simulink model "gm_CustArch_v5_vnl"  (R2020a)
settings: Solver=FixedStepDiscrete  StartTime=0.0  StopTime=840000  RelTol=1e-3
libraries: simulink x179, hdlsllib x113
(part 3 of 4)

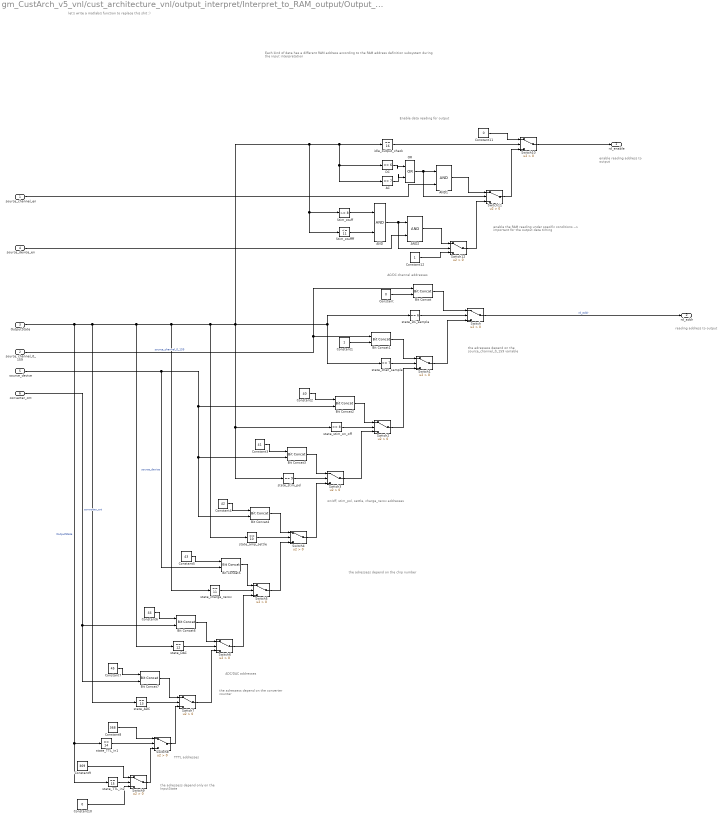
== system gm_CustArch_v5_vnl/cust_architecture_vnl/output_interpret/Interpret_to_RAM_output/Output_State_to_RAM_address (to read) ==
  note: enable reading address
      | to output
  note: Each kind of data has a different RAM
      | address according to the
      | RAM address definition subsystem during the
      | input interpretation
  note: the adressess depend on the
      | source_channel_0_159 variable
  note: AC/DC channel addresses
  note: ADC/DAC addresses
  note: on/off, stim_pol, settle, charge_recov addresses
  note: the adressess depend on the converter
      | counter
  note: the adressess depend only on the
      | InputState
  note: the adressess depend on the chip number
  note: TTTL addresses
  note: let's write a matlab/s function to replace this shit :)
  note: Enable data reading for output
  note: enable the RAM reading under specific conditions
      | --> important for the output data timing
  note: reading address
      | to output
  source_channel_en : Inport
  source_channel_0_159 : Inport  Port=2
  OutputState : Inport  Port=3
  source_device_en : Inport  Port=4
  source_device : Inport  Port=5
  converter_cnt : Inport  Port=6
  AC : simulink/Logic and Bit Operations/Compare To Constant  relop===  const=7  OutDataTypeStr=boolean
  AND : Logic  IconShape=distinctive  AllPortsSameDT=off  OutDataTypeStr=boolean
  AND1 : Logic  IconShape=distinctive  AllPortsSameDT=off  OutDataTypeStr=boolean
  AND2 : Logic  IconShape=distinctive  AllPortsSameDT=off  OutDataTypeStr=boolean
  Bit Concat{,1..7} (8 alike) : hdlsllib/Logic and Bit Operations/Bit Concat  numInputs=2
  Constant : Constant  Value=0  OutDataTypeStr=boolean  SampleTime=-1
  Constant1 : Constant  OutDataTypeStr=boolean  SampleTime=-1
  Constant10 : Constant  Value=0  OutDataTypeStr=fixdt(0,9)  SampleTime=-1
  Constant11 : Constant  Value=0  OutDataTypeStr=boolean  SampleTime=-1
  Constant12 : Constant  OutDataTypeStr=boolean  SampleTime=-1
  Constant2 : Constant  Value=40  OutDataTypeStr=fixdt(0,6)  SampleTime=-1
  Constant3 : Constant  Value=41  OutDataTypeStr=fixdt(0,6)  SampleTime=-1
  Constant4 : Constant  Value=42  OutDataTypeStr=fixdt(0,6)  SampleTime=-1
  Constant5 : Constant  Value=43  OutDataTypeStr=fixdt(0,6)  SampleTime=-1
  Constant6 : Constant  Value=44  OutDataTypeStr=fixdt(0,6)  SampleTime=-1
  Constant7 : Constant  Value=45  OutDataTypeStr=fixdt(0,6)  SampleTime=-1
  Constant8 : Constant  Value=368  OutDataTypeStr=fixdt(0,9)  SampleTime=-1
  Constant9 : Constant  Value=369  OutDataTypeStr=fixdt(0,9)  SampleTime=-1
  DC : simulink/Logic and Bit Operations/Compare To Constant  relop===  const=6  OutDataTypeStr=boolean
  OR : Logic  Operator=OR  IconShape=distinctive  AllPortsSameDT=off  OutDataTypeStr=boolean
  Stim_stuff : simulink/Logic and Bit Operations/Compare To Constant  relop=>=  const=8  OutDataTypeStr=boolean
  Stim_stuffff : simulink/Logic and Bit Operations/Compare To Constant  relop=<=  const=11  OutDataTypeStr=boolean
  Switch{,1..12} (13 alike) : Switch  Criteria=u2 > Threshold
  idle_output_check : simulink/Logic and Bit Operations/Compare To Constant  relop===  const=16  OutDataTypeStr=boolean
  state_ADC : simulink/Logic and Bit Operations/Compare To Constant  relop===  const=13  OutDataTypeStr=boolean
  state_DAC : simulink/Logic and Bit Operations/Compare To Constant  relop===  const=12  OutDataTypeStr=boolean
  state_DC_sample : simulink/Logic and Bit Operations/Compare To Constant  relop===  const=6  OutDataTypeStr=boolean
  state_TTL_in1 : simulink/Logic and Bit Operations/Compare To Constant  relop===  const=14  OutDataTypeStr=boolean
  state_TTL_in2 : simulink/Logic and Bit Operations/Compare To Constant  relop===  const=15  OutDataTypeStr=boolean
  state_amp_settle : simulink/Logic and Bit Operations/Compare To Constant  relop===  const=10  OutDataTypeStr=boolean
  state_chan_sample : simulink/Logic and Bit Operations/Compare To Constant  relop===  const=7  OutDataTypeStr=boolean
  state_charge_recov : simulink/Logic and Bit Operations/Compare To Constant  relop===  const=11  OutDataTypeStr=boolean
  state_stim_on_off : simulink/Logic and Bit Operations/Compare To Constant  relop===  const=8  OutDataTypeStr=boolean
  state_stim_pol : simulink/Logic and Bit Operations/Compare To Constant  relop===  const=9  OutDataTypeStr=boolean
  rd_enable : Outport  VectorParamsAs1DForOutWhenUnconnected=off
  rd_addr : Outport  Port=2  OutDataTypeStr=fixdt(0,9,0)  VectorParamsAs1DForOutWhenUnconnected=off
  wires:
  Switch10/1 -> rd_enable/1
  Constant12/1 -> Switch12/3
  Switch12/1 -> Switch11/3
  AND2/1 -> Switch12/1
  AND1/1 -> Switch11/1
  Switch11/1 -> Switch10/3
  Constant11/1 -> Switch10/1
  source_device_en/1 -> AND2/2
  source_channel_en/1 -> AND1/2
  AND/1 -> AND2/1, Switch12/2
  Stim_stuffff/1 -> AND/2
  Stim_stuff/1 -> AND/1
  idle_output_check/1 -> Switch10/2
  OR/1 -> AND1/1, Switch11/2
  AC/1 -> OR/2
  DC/1 -> OR/1
  Constant10/1 -> Switch9/3
  Switch9/1 -> Switch8/3
  Constant9/1 -> Switch9/1
  state_TTL_in2/1 -> Switch9/2
  Switch8/1 -> Switch7/3
  OutputState/1 -> state_ADC/1, state_charge_recov/1, Stim_stuff/1, Stim_stuffff/1, idle_output_check/1, DC/1, AC/1, state_chan_sample/1, state_DC_sample/1, state_stim_on_off/1, state_stim_pol/1, state_amp_settle/1, state_DAC/1, state_TTL_in1/1, state_TTL_in2/1  "OutputState"
  Constant8/1 -> Switch8/1
  state_TTL_in1/1 -> Switch8/2
  Switch7/1 -> Switch6/3
  Constant7/1 -> Bit Concat7/1
  state_ADC/1 -> Switch7/2
  Bit Concat7/1 -> Switch7/1
  converter_cnt/1 -> Bit Concat6/2, Bit Concat7/2  "converter_cnt"
  Switch6/1 -> Switch5/3
  Constant6/1 -> Bit Concat6/1
  state_DAC/1 -> Switch6/2
  Bit Concat6/1 -> Switch6/1
  Switch5/1 -> Switch4/3
  source_device/1 -> Bit Concat2/2, Bit Concat3/2, Bit Concat4/2, Bit Concat5/2  "source_device"
  Constant5/1 -> Bit Concat5/1
  state_charge_recov/1 -> Switch5/2
  Bit Concat5/1 -> Switch5/1
  Switch4/1 -> Switch3/3
  Bit Concat4/1 -> Switch4/1
  state_amp_settle/1 -> Switch4/2
  Constant4/1 -> Bit Concat4/1
  Switch3/1 -> Switch2/3
  Bit Concat3/1 -> Switch3/1
  state_stim_pol/1 -> Switch3/2
  Constant3/1 -> Bit Concat3/1
  Switch2/1 -> Switch1/3
  state_stim_on_off/1 -> Switch2/2
  Bit Concat2/1 -> Switch2/1
  Constant2/1 -> Bit Concat2/1
  Switch/1 -> rd_addr/1  "rd_addr"
  Switch1/1 -> Switch/3
  Bit Concat1/1 -> Switch1/1
  Constant1/1 -> Bit Concat1/2
  state_chan_sample/1 -> Switch1/2
  Bit Concat/1 -> Switch/1
  Constant/1 -> Bit Concat/2
  source_channel_0_159/1 -> Bit Concat/1, Bit Concat1/1  "source_channel_0_159"
  state_DC_sample/1 -> Switch/2

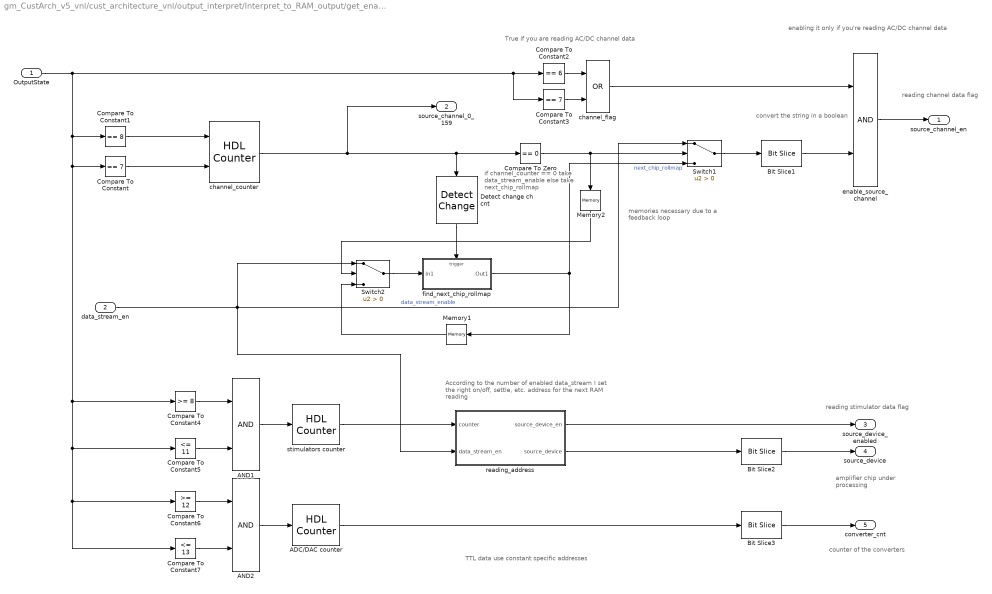
== system gm_CustArch_v5_vnl/cust_architecture_vnl/output_interpret/Interpret_to_RAM_output/get_enabled_timings  ==
  note: counter of the converters
  note: reading stimulator data flag
  note: TTL data use constant specific addresses
  note: enabling it only if you're reading AC/DC channel data
  note: True if you are reading AC/DC channel data
  note: convert the string
      | in a boolean
  note: According to the number of enabled data_stream
      | I set the right on/off, settle, etc. address for the next
      | RAM reading
  note: amplifier chip under
      | processing
  note: if channel_counter == 0
      | take data_stream_enable
      | else take next_chip_rollmap
  note: memories necessary due to
      | a feedback loop
  note: reading channel data flag
  OutputState : Inport
  data_stream_en : Inport  Port=2
  ADC/DAC counter : hdlsllib/Sources/HDL Counter  CountType=Count limited  CountInit=0  CountStep=1  CountMax=7  CountFromType=Specify  CountFrom=0  CountResetPort=off  CountLoadPort=off  CountEnbPort=on  CountDirPort=off  CountDataType=Unsigned  CountWordLen=8  CountFracLen=0  CountSampTime=1
  AND1 : Logic  IconShape=distinctive  AllPortsSameDT=off  OutDataTypeStr=boolean
  AND2 : Logic  IconShape=distinctive  AllPortsSameDT=off  OutDataTypeStr=boolean
  Bit Slice1 : hdlsllib/Logic and Bit Operations/Bit Slice  lidx=0  ridx=0
      settings: SourceProductBaseCode=SL
  Bit Slice2 : hdlsllib/Logic and Bit Operations/Bit Slice  lidx=2  ridx=0
      settings: SourceProductBaseCode=SL
  Bit Slice3 : hdlsllib/Logic and Bit Operations/Bit Slice  lidx=2  ridx=0
      settings: SourceProductBaseCode=SL
  Compare To Constant : simulink/Logic and Bit Operations/Compare To Constant  relop===  const=7  OutDataTypeStr=boolean
  Compare To Constant1 : simulink/Logic and Bit Operations/Compare To Constant  relop===  const=8  OutDataTypeStr=boolean
  Compare To Constant2 : simulink/Logic and Bit Operations/Compare To Constant  relop===  const=6  OutDataTypeStr=boolean
  Compare To Constant3 : simulink/Logic and Bit Operations/Compare To Constant  relop===  const=7  OutDataTypeStr=boolean
  Compare To Constant4 : simulink/Logic and Bit Operations/Compare To Constant  relop=>=  const=8  OutDataTypeStr=boolean
  Compare To Constant5 : simulink/Logic and Bit Operations/Compare To Constant  relop=<=  const=11  OutDataTypeStr=boolean
  Compare To Constant6 : simulink/Logic and Bit Operations/Compare To Constant  relop=>=  const=12  OutDataTypeStr=boolean
  Compare To Constant7 : simulink/Logic and Bit Operations/Compare To Constant  relop=<=  const=13  OutDataTypeStr=boolean
  Compare To Zero : simulink/Logic and Bit Operations/Compare To Zero  relop===  OutDataTypeStr=boolean
  Detect change ch cnt : simulink/Logic and Bit Operations/Detect Change  vinit=0  OutDataTypeStr=boolean
  Memory1 : Memory  InheritSampleTime=on
  Memory2 : Memory  InheritSampleTime=on
  Switch1 : Switch  Criteria=u2 > Threshold
  Switch2 : Switch  Criteria=u2 > Threshold
  channel_counter : hdlsllib/Sources/HDL Counter  CountType=Count limited  CountInit=0  CountStep=1  CountMax=159  CountFromType=Specify  CountFrom=0  CountResetPort=on  CountLoadPort=off  CountEnbPort=on  CountDirPort=off  CountDataType=Unsigned  CountWordLen=8  CountFracLen=0  CountSampTime=1
  channel_flag : Logic  Operator=OR  IconShape=distinctive  AllPortsSameDT=off  OutDataTypeStr=boolean
  enable_source_channel : Logic  IconShape=distinctive  AllPortsSameDT=off  OutDataTypeStr=boolean
  find_next_chip_rollmap : Subsystem  TreatAsAtomicUnit=on
  reading_address : Subsystem
  stimulators counter : hdlsllib/Sources/HDL Counter  CountType=Count limited  CountInit=0  CountStep=1  CountMax=7  CountFromType=Specify  CountFrom=0  CountResetPort=off  CountLoadPort=off  CountEnbPort=on  CountDirPort=off  CountDataType=Unsigned  CountWordLen=8  CountFracLen=0  CountSampTime=1
  source_channel_en : Outport  VectorParamsAs1DForOutWhenUnconnected=off
  source_channel_0_159 : Outport  Port=2  OutMin=0  OutMax=159  OutDataTypeStr=uint8  VectorParamsAs1DForOutWhenUnconnected=off  LockScale=on
  source_device_enabled : Outport  Port=3  VectorParamsAs1DForOutWhenUnconnected=off
  source_device : Outport  Port=4  VectorParamsAs1DForOutWhenUnconnected=off
  converter_cnt : Outport  Port=5  VectorParamsAs1DForOutWhenUnconnected=off
  wires:
  Compare To Constant/1 -> channel_counter/2
  Compare To Constant1/1 -> channel_counter/1
  ADC/DAC counter/1 -> Bit Slice3/1
  AND2/1 -> ADC/DAC counter/1
  Compare To Constant7/1 -> AND2/2
  OutputState/1 -> Compare To Constant2/1, Compare To Constant3/1, Compare To Constant4/1, Compare To Constant5/1, Compare To Constant7/1, Compare To Constant6/1, Compare To Constant/1, Compare To Constant1/1
  Bit Slice3/1 -> converter_cnt/1
  Compare To Constant6/1 -> AND2/1
  data_stream_en/1 -> Switch2/1, reading_address/2(data_stream_en), Switch1/1  "data_stream_enable"
  reading_address/2(source_device) -> Bit Slice2/1
  stimulators counter/1 -> reading_address/1("counter ")
  AND1/1 -> stimulators counter/1
  Bit Slice2/1 -> source_device/1
  reading_address/1(source_device_en) -> source_device_enabled/1
  Compare To Constant5/1 -> AND1/2
  Compare To Constant4/1 -> AND1/1
  Bit Slice1/1 -> enable_source_channel/2
  Switch1/1 -> Bit Slice1/1
  enable_source_channel/1 -> source_channel_en/1
  channel_flag/1 -> enable_source_channel/1
  Compare To Constant2/1 -> channel_flag/1
  Compare To Constant3/1 -> channel_flag/2
  Memory2/1 -> Switch2/2
  Compare To Zero/1 -> Memory2/1, Switch1/2
  Switch2/1 -> find_next_chip_rollmap/1(In1)
  Memory1/1 -> Switch2/3
  find_next_chip_rollmap/1(Out1) -> Switch1/3, Memory1/1  "next_chip_rollmap"
  Detect change ch cnt/1 -> find_next_chip_rollmap/Trigger
  channel_counter/1 -> source_channel_0_159/1, Compare To Zero/1, Detect change ch cnt/1

== system gm_CustArch_v5_vnl/cust_architecture_vnl/process_and_retrieve/digital_filter/HP_Butter_1st ==
  Input : Inport  OutDataTypeStr=fixdt(1,16,4)
  Input1 : Inport  Port=2  OutDataTypeStr=fixdt(1,16,2)
  CastState1 : DataTypeConversion  OutDataTypeStr=fixdt(1,16,2)  RndMeth=Convergent  SaturateOnIntegerOverflow=on
  ConvertIn : DataTypeConversion  OutDataTypeStr=fixdt(1,16,4)  RndMeth=Nearest  SaturateOnIntegerOverflow=on
  ConvertOut : DataTypeConversion  OutDataTypeStr=fixdt(1,16,5)  RndMeth=Convergent  SaturateOnIntegerOverflow=on
  SumA21 : Sum  Inputs=|+-  AccumDataTypeStr=fixdt(1,34,20)  OutDataTypeStr=fixdt(1,34,20)  RndMeth=Convergent  SaturateOnIntegerOverflow=on
  SumB21 : Sum  Inputs=|+-  AccumDataTypeStr=fixdt(1,34,20)  OutDataTypeStr=fixdt(1,34,23)  RndMeth=Convergent  SaturateOnIntegerOverflow=on
  a(2)(1) : Gain  Gain=-0.939062505817492399  ParamDataTypeStr=fixdt(1,16,15)  OutDataTypeStr=fixdt(1,32,18)  RndMeth=Convergent  SaturateOnIntegerOverflow=on
  s(1) : Gain  Gain=0.969531252908746199  ParamDataTypeStr=fixdt(0,16,16)  OutDataTypeStr=fixdt(1,16,4)  RndMeth=Convergent  SaturateOnIntegerOverflow=on
  Output : Outport
  Output1 : Outport  Port=2
  wires:
  Input1/1 -> a(2)(1)/1, SumB21/2
  ConvertIn/1 -> s(1)/1
  ConvertOut/1 -> Output/1
  CastState1/1 -> SumB21/1, Output1/1
  a(2)(1)/1 -> SumA21/2
  SumB21/1 -> ConvertOut/1
  SumA21/1 -> CastState1/1
  s(1)/1 -> SumA21/1
  Input/1 -> ConvertIn/1

== system gm_CustArch_v5_vnl/cust_architecture_vnl/process_and_retrieve/previous_sample_storage/PreviousData_read ==
  u2 : Inport
  Enable : EnablePort
  1st1 : Constant  OutDataTypeStr=boolean  SampleTime=-1
  Bit Concat1 : hdlsllib/Logic and Bit Operations/Bit Concat  numInputs=2
  y : Outport  InitialOutput=[0]
  wires:
  Bit Concat1/1 -> y/1
  1st1/1 -> Bit Concat1/1
  u2/1 -> Bit Concat1/2

== system gm_CustArch_v5_vnl/cust_architecture_vnl/process_and_retrieve/previous_sample_storage1/PreviousData_read ==
  u2 : Inport
  Enable : EnablePort  StatesWhenEnabling=reset
  1st1 : Constant  OutDataTypeStr=boolean  SampleTime=-1
  Bit Concat1 : hdlsllib/Logic and Bit Operations/Bit Concat  numInputs=2
  y : Outport  OutputWhenDisabled=reset  InitialOutput=[0]
  wires:
  Bit Concat1/1 -> y/1
  1st1/1 -> Bit Concat1/1
  u2/1 -> Bit Concat1/2

== system gm_CustArch_v5_vnl/cust_architecture/input_interpret_store_retrieve/Interpret_to_RAM_input/interpret incoming data/condition to count DAC or ADC  ==
  fifo_write_to : Inport  OutDataTypeStr=boolean  PortDimensions=1  SampleTime=1
  input_state : Inport  Port=2  OutDataTypeStr=uint8  PortDimensions=1  SampleTime=1
  AND : Logic  AllPortsSameDT=off  OutDataTypeStr=boolean  SampleTime=1
  OR : Logic  Operator=OR  AllPortsSameDT=off  OutDataTypeStr=boolean  SampleTime=1
  is state_ADC : simulink/Logic and Bit Operations/Compare To Constant  relop===  const="fi(0,0,8,0,\"hex\",\"0d\")"  OutDataTypeStr=boolean
  is state_DAC : simulink/Logic and Bit Operations/Compare To Constant  relop===  const="fi(0,0,8,0,\"hex\",\"0c\")"  OutDataTypeStr=boolean
  Out1 : Outport  VectorParamsAs1DForOutWhenUnconnected=off
  wires:
  is state_DAC/1 -> OR/1
  is state_ADC/1 -> OR/2
  OR/1 -> AND/2
  AND/1 -> Out1/1
  input_state/1 -> is state_ADC/1, is state_DAC/1
  fifo_write_to/1 -> AND/1

== system gm_CustArch_v5_vnl/cust_architecture/input_interpret_store_retrieve/Interpret_to_RAM_input/interpret incoming data/get_sources_and_RAM_addresses ==
  note: necessary to move forward from state 6 to 8
  note: 0-159 --> 20 (16 electrodes + 4 aux commands) x 8 chips
  note: if next_chip_rollmap == 00000000 I have cycled among all the chip so let's restart from data_stream_enable
  note: the data_stream_enable is a 8-bit string in which if a bit is 1 the data stream of that chip is enabled
  note: TTL data use constant specific addresses
  FIFO_write_to : Inport  OutDataTypeStr=boolean  PortDimensions=1  SampleTime=1
  InputState : Inport  Port=2  OutDataTypeStr=uint8  PortDimensions=1  SampleTime=1
  data_stream_enable : Inport  Port=3  OutDataTypeStr=uint8  PortDimensions=1  SampleTime=1
  AND1 : Logic  AllPortsSameDT=off  OutDataTypeStr=boolean  SampleTime=1
  AND2 : Logic  AllPortsSameDT=off  OutDataTypeStr=boolean  SampleTime=1
  AND3 : Logic  AllPortsSameDT=off  OutDataTypeStr=boolean  SampleTime=1
  Compare To Constant1 : simulink/Logic and Bit Operations/Compare To Constant  relop===  const="fi(0,0,8,0,\"hex\",\"00\")"  OutDataTypeStr=boolean
  Compare To Constant2 : simulink/Logic and Bit Operations/Compare To Constant  relop===  const="fi(0,0,8,0,\"hex\",\"0d\")"  OutDataTypeStr=boolean
  Compare To Constant3 : simulink/Logic and Bit Operations/Compare To Constant  relop===  const="fi(0,0,8,0,\"hex\",\"06\")"  OutDataTypeStr=boolean
  Compare To Constant4 : simulink/Logic and Bit Operations/Compare To Constant  relop=>=  const="fi(0,0,8,0,\"hex\",\"08\")"  OutDataTypeStr=boolean
  Compare To Constant5 : simulink/Logic and Bit Operations/Compare To Constant  relop===  const="fi(0,0,8,0,\"hex\",\"00\")"  OutDataTypeStr=boolean
  Compare To Constant6 : simulink/Logic and Bit Operations/Compare To Constant  relop=<=  const="fi(0,0,8,0,\"hex\",\"0b\")"  OutDataTypeStr=boolean
  Memory : UnitDelay  InitialCondition=double(0)  SampleTime=1
  Memory1 : UnitDelay  InitialCondition=double(0)  SampleTime=1
  Memory2 : UnitDelay  InitialCondition=double(0)  SampleTime=1
  OR : Logic  Operator=OR  AllPortsSameDT=off  OutDataTypeStr=boolean  SampleTime=1
  RAM_address_channel_data : Subsystem
  Switch : Switch  Criteria=u2 > Threshold  Threshold=double(0)  OutDataTypeStr=uint8  SampleTime=1
  Switch1 : Switch  Criteria=u2 > Threshold  Threshold=double(0)  OutDataTypeStr=uint8  SampleTime=1
  channel_counter : hdlsllib/Sources/HDL Counter  CountType=Count limited  CountInit=double(0)  CountStep=double(1)  CountMax=double(20)  CountFromType=Initial value  CountFrom=double(0)  CountResetPort=on  CountLoadPort=off  CountEnbPort=on  CountDirPort=off  CountDataType=Unsigned  CountWordLen=8  CountFracLen=0  CountSampTime=1
  enable_RAM_indexing : Logic  AllPortsSameDT=off  OutDataTypeStr=boolean  SampleTime=1
  enable_source_chip_transmission : Subsystem
  find_first_one_pos : Subsystem
  find_next_chip_rollmap : Subsystem
  source_device : Outport  VectorParamsAs1DForOutWhenUnconnected=off
  device_output : Outport  Port=2  VectorParamsAs1DForOutWhenUnconnected=off
  source_channel : Outport  Port=3  VectorParamsAs1DForOutWhenUnconnected=off
  inc_source_device : Outport  Port=4  VectorParamsAs1DForOutWhenUnconnected=off
  wires:
  find_next_chip_rollmap/1(bit_masked) -> Memory/1, Compare To Constant5/1
  find_first_one_pos/1(first_one_pos) -> find_next_chip_rollmap/2(source_chip), enable_source_chip_transmission/1(In1)
  enable_source_chip_transmission/1(Out1) -> RAM_address_channel_data/1(source_device), source_device/1
  enable_RAM_indexing/1 -> find_first_one_pos/Enable, find_next_chip_rollmap/Enable, RAM_address_channel_data/Enable, enable_source_chip_transmission/Enable, Memory2/1, AND2/1
  channel_counter/1 -> RAM_address_channel_data/2(dev_output), device_output/1
  Switch1/1 -> Switch/3
  Switch/1 -> find_first_one_pos/1(In1), find_next_chip_rollmap/1(curr_chip_rollmap)
  RAM_address_channel_data/1(source_channel_0_159) -> source_channel/1
  OR/1 -> enable_RAM_indexing/2
  Memory2/1 -> AND3/2
  Memory1/1 -> AND3/1, Switch1/2
  Memory/1 -> Switch1/3
  Compare To Constant6/1 -> AND1/2
  Compare To Constant5/1 -> Memory1/1, AND2/2
  Compare To Constant4/1 -> AND1/1
  Compare To Constant3/1 -> OR/1
  Compare To Constant2/1 -> channel_counter/1
  Compare To Constant1/1 -> Switch/2
  AND3/1 -> channel_counter/2
  AND2/1 -> inc_source_device/1
  AND1/1 -> OR/2
  data_stream_enable/1 -> Switch/1, Switch1/1
  InputState/1 -> Compare To Constant1/1, Compare To Constant2/1, Compare To Constant3/1, Compare To Constant4/1, Compare To Constant6/1
  FIFO_write_to/1 -> enable_RAM_indexing/1

== system gm_CustArch_v5_vnl/cust_architecture/output_interpret/Interpret_to_RAM_output/get_enabled_timings /find_next_chip_rollmap ==
  In1 : Inport  OutDataTypeStr=uint8  PortDimensions=1
  Trigger : TriggerPort  VariantControl=(inherit)  PortDimensions=1  OutDataTypeStr=boolean
  Bit Rotate : hdlsllib/Logic and Bit Operations/Bit Rotate  mode=Rotate Right  N=double(1)
      settings: SourceProductBaseCode=SL
  Out1 : Outport  InitialOutput=0  VectorParamsAs1DForOutWhenUnconnected=off
  wires:
  Bit Rotate/1 -> Out1/1
  In1/1 -> Bit Rotate/1

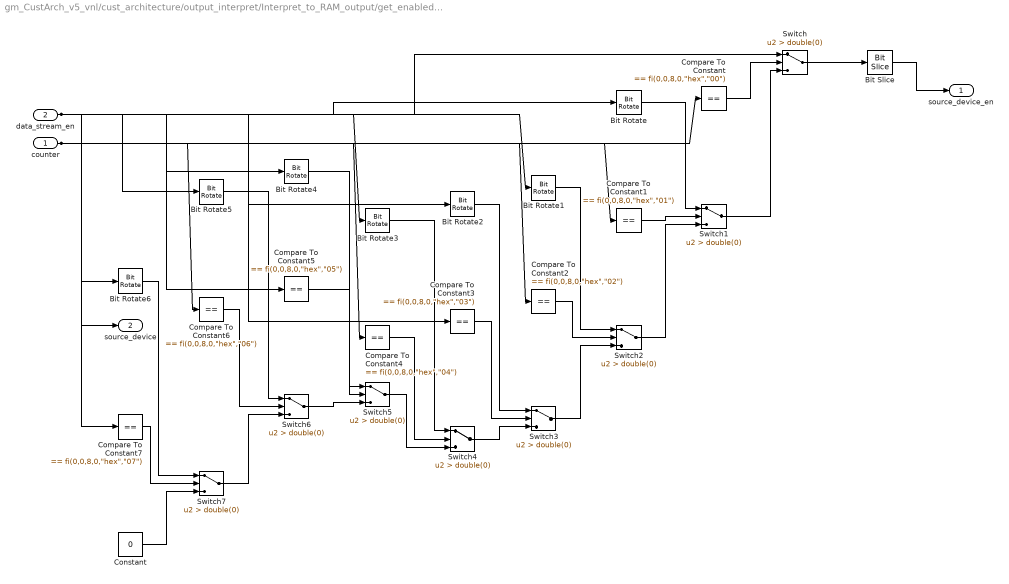
== system gm_CustArch_v5_vnl/cust_architecture/output_interpret/Interpret_to_RAM_output/get_enabled_timings /reading_address ==
  "counter " : Inport  OutDataTypeStr=uint8  PortDimensions=1  SampleTime=1
  data_stream_en : Inport  Port=2  OutDataTypeStr=uint8  PortDimensions=1  SampleTime=1
  Bit Rotate : hdlsllib/Logic and Bit Operations/Bit Rotate  mode=Rotate Right  N=double(1)
      settings: SourceProductBaseCode=SL
  Bit Rotate1 : hdlsllib/Logic and Bit Operations/Bit Rotate  mode=Rotate Right  N=double(2)
      settings: SourceProductBaseCode=SL
  Bit Rotate2 : hdlsllib/Logic and Bit Operations/Bit Rotate  mode=Rotate Right  N=double(3)
      settings: SourceProductBaseCode=SL
  Bit Rotate3 : hdlsllib/Logic and Bit Operations/Bit Rotate  mode=Rotate Right  N=double(4)
      settings: SourceProductBaseCode=SL
  Bit Rotate4 : hdlsllib/Logic and Bit Operations/Bit Rotate  mode=Rotate Right  N=double(5)
      settings: SourceProductBaseCode=SL
  Bit Rotate5 : hdlsllib/Logic and Bit Operations/Bit Rotate  mode=Rotate Right  N=double(6)
      settings: SourceProductBaseCode=SL
  Bit Rotate6 : hdlsllib/Logic and Bit Operations/Bit Rotate  mode=Rotate Right  N=double(7)
      settings: SourceProductBaseCode=SL
  Bit Slice : hdlsllib/Logic and Bit Operations/Bit Slice  lidx=double(0)  ridx=double(0)
      settings: SourceProductBaseCode=SL
  Compare To Constant : simulink/Logic and Bit Operations/Compare To Constant  relop===  const="fi(0,0,8,0,\"hex\",\"00\")"  OutDataTypeStr=boolean
  Compare To Constant1 : simulink/Logic and Bit Operations/Compare To Constant  relop===  const="fi(0,0,8,0,\"hex\",\"01\")"  OutDataTypeStr=boolean
  Compare To Constant2 : simulink/Logic and Bit Operations/Compare To Constant  relop===  const="fi(0,0,8,0,\"hex\",\"02\")"  OutDataTypeStr=boolean
  Compare To Constant3 : simulink/Logic and Bit Operations/Compare To Constant  relop===  const="fi(0,0,8,0,\"hex\",\"03\")"  OutDataTypeStr=boolean
  Compare To Constant4 : simulink/Logic and Bit Operations/Compare To Constant  relop===  const="fi(0,0,8,0,\"hex\",\"04\")"  OutDataTypeStr=boolean
  Compare To Constant5 : simulink/Logic and Bit Operations/Compare To Constant  relop===  const="fi(0,0,8,0,\"hex\",\"05\")"  OutDataTypeStr=boolean
  Compare To Constant6 : simulink/Logic and Bit Operations/Compare To Constant  relop===  const="fi(0,0,8,0,\"hex\",\"06\")"  OutDataTypeStr=boolean
  Compare To Constant7 : simulink/Logic and Bit Operations/Compare To Constant  relop===  const="fi(0,0,8,0,\"hex\",\"07\")"  OutDataTypeStr=boolean
  Constant : Constant  Value=0  OutDataTypeStr=uint8  SampleTime=1
  Switch{,1..7} (8 alike) : Switch  Criteria=u2 > Threshold  Threshold=double(0)  OutDataTypeStr=uint8  SampleTime=1
  source_device_en : Outport  VectorParamsAs1DForOutWhenUnconnected=off
  source_device : Outport  Port=2  VectorParamsAs1DForOutWhenUnconnected=off
  wires:
  Switch7/1 -> Switch6/3
  Switch6/1 -> Switch5/3
  Switch5/1 -> Switch4/3
  Switch4/1 -> Switch3/3
  Switch3/1 -> Switch2/3
  Switch2/1 -> Switch1/3
  Switch1/1 -> Switch/3
  Switch/1 -> Bit Slice/1
  Constant/1 -> Switch7/3
  Compare To Constant7/1 -> Switch7/2
  Compare To Constant6/1 -> Switch6/2
  Compare To Constant5/1 -> Switch5/2
  Compare To Constant4/1 -> Switch4/2
  Compare To Constant3/1 -> Switch3/2
  Compare To Constant2/1 -> Switch2/2
  Compare To Constant1/1 -> Switch1/2
  Compare To Constant/1 -> Switch/2
  Bit Slice/1 -> source_device_en/1
  Bit Rotate6/1 -> Switch7/1
  Bit Rotate5/1 -> Switch6/1
  Bit Rotate4/1 -> Switch5/1
  Bit Rotate3/1 -> Switch4/1
  Bit Rotate2/1 -> Switch3/1
  Bit Rotate1/1 -> Switch2/1
  Bit Rotate/1 -> Switch1/1
  data_stream_en/1 -> Bit Rotate/1, Bit Rotate1/1, Bit Rotate2/1, Bit Rotate3/1, Bit Rotate4/1, Bit Rotate5/1, Bit Rotate6/1, Switch/1
  "counter "/1 -> source_device/1, Compare To Constant/1, Compare To Constant1/1, Compare To Constant2/1, Compare To Constant3/1, Compare To Constant4/1, Compare To Constant5/1, Compare To Constant6/1, Compare To Constant7/1

== system gm_CustArch_v5_vnl/cust_architecture_vnl/input_interpret_store_retrieve/Interpret_to_RAM_input/interpret incoming data/condition to count DAC or ADC  ==
  fifo_write_to : Inport
  input_state : Inport  Port=2
  AND : Logic  IconShape=distinctive  AllPortsSameDT=off  OutDataTypeStr=boolean
  OR : Logic  Operator=OR  IconShape=distinctive  AllPortsSameDT=off  OutDataTypeStr=boolean
  is state_ADC : simulink/Logic and Bit Operations/Compare To Constant  relop===  const=13  OutDataTypeStr=boolean
  is state_DAC : simulink/Logic and Bit Operations/Compare To Constant  relop===  const=12  OutDataTypeStr=boolean
  Out1 : Outport  VectorParamsAs1DForOutWhenUnconnected=off
  wires:
  AND/1 -> Out1/1
  OR/1 -> AND/2
  fifo_write_to/1 -> AND/1
  is state_ADC/1 -> OR/2
  is state_DAC/1 -> OR/1
  input_state/1 -> is state_ADC/1, is state_DAC/1

== system gm_CustArch_v5_vnl/cust_architecture_vnl/input_interpret_store_retrieve/Interpret_to_RAM_input/interpret incoming data/get_sources_and_RAM_addresses ==
  note: TTL data use constant specific addresses
  note: channel data
      | address
  note: channel (electrode) under
      | processing
  note: the data_stream_enable is a 8-bit string in which if a bit is 1 the data stream of that chip is enabled
  note: if next_chip_rollmap == 00000000 I have cycled among all the chip so let's restart from data_stream_enable
  note: to identify the first position in which
      | I am able to find a 1
  note: 0-159 --> 20 (16 electrodes + 4 aux commands) x 8 chips
  note: if InputState == 0 (starting state corresponding to the first byte
      | of the magic number) the data_stream_enable goes through the switch
  note: whether or not enable the address definition
      | for the RAM writing
  note: if InputState == 13
      | reset the channel counter
  note: the channel_counter increments the
      | device_output variable every time the
      | current_chip rollmap is equal to 00000000
      | (rollmap concluded)
  note: amplifier chip under
      | processing
  note: necessary to move forward from state 6 to 8
  FIFO_write_to : Inport
  InputState : Inport  Port=2
  data_stream_enable : Inport  Port=3
  AND1 : Logic  IconShape=distinctive  AllPortsSameDT=off  OutDataTypeStr=boolean
  AND2 : Logic  IconShape=distinctive  AllPortsSameDT=off  OutDataTypeStr=boolean
  AND3 : Logic  IconShape=distinctive  AllPortsSameDT=off  OutDataTypeStr=boolean
  Compare To Constant1 : simulink/Logic and Bit Operations/Compare To Constant  relop===  const=0  OutDataTypeStr=boolean
  Compare To Constant2 : simulink/Logic and Bit Operations/Compare To Constant  relop===  const=13  OutDataTypeStr=boolean
  Compare To Constant3 : simulink/Logic and Bit Operations/Compare To Constant  relop===  const=6  OutDataTypeStr=boolean
  Compare To Constant4 : simulink/Logic and Bit Operations/Compare To Constant  relop=>=  const=8  OutDataTypeStr=boolean
  Compare To Constant5 : simulink/Logic and Bit Operations/Compare To Constant  relop===  const=0  OutDataTypeStr=boolean
  Compare To Constant6 : simulink/Logic and Bit Operations/Compare To Constant  relop=<=  const=11  OutDataTypeStr=boolean
  Memory : Memory  InheritSampleTime=on
  Memory1 : Memory  InheritSampleTime=on
  Memory2 : Memory  InheritSampleTime=on
  OR : Logic  Operator=OR  IconShape=distinctive  AllPortsSameDT=off  OutDataTypeStr=boolean
  RAM_address_channel_data : Subsystem
  Switch : Switch  Criteria=u2 > Threshold  OutDataTypeStr=uint8
  Switch1 : Switch  Criteria=u2 > Threshold
  channel_counter : hdlsllib/Sources/HDL Counter  CountType=Count limited  CountInit=0  CountStep=1  CountMax=20  CountFromType=Specify  CountFrom=0  CountResetPort=on  CountLoadPort=off  CountEnbPort=on  CountDirPort=off  CountDataType=Unsigned  CountWordLen=8  CountFracLen=0  CountSampTime=1
  enable_RAM_indexing : Logic  IconShape=distinctive  AllPortsSameDT=off  OutDataTypeStr=boolean
  enable_source_chip_transmission : Subsystem  TreatAsAtomicUnit=on
  find_first_one_pos : Subsystem
  find_next_chip_rollmap : Subsystem
  source_device : Outport  VectorParamsAs1DForOutWhenUnconnected=off
  device_output : Outport  Port=2  VectorParamsAs1DForOutWhenUnconnected=off
  source_channel : Outport  Port=3  VectorParamsAs1DForOutWhenUnconnected=off
  inc_source_device : Outport  Port=4  VectorParamsAs1DForOutWhenUnconnected=off
  wires:
  find_first_one_pos/1(first_one_pos) -> find_next_chip_rollmap/2(source_chip), enable_source_chip_transmission/1(In1)  "source_device"
  AND2/1 -> inc_source_device/1
  Memory1/1 -> Switch1/2, AND3/1
  OR/1 -> enable_RAM_indexing/2
  AND1/1 -> OR/2
  Compare To Constant6/1 -> AND1/2
  Compare To Constant4/1 -> AND1/1
  Compare To Constant2/1 -> channel_counter/1
  RAM_address_channel_data/1(source_channel_0_159) -> source_channel/1  "source_channel_0_159"
  Compare To Constant3/1 -> OR/1
  enable_source_chip_transmission/1(Out1) -> RAM_address_channel_data/1(source_device), source_device/1  "source_device"
  Memory2/1 -> AND3/2
  Memory/1 -> Switch1/3
  AND3/1 -> channel_counter/2
  channel_counter/1 -> RAM_address_channel_data/2(dev_output), device_output/1  "device_output"
  Compare To Constant5/1 -> Memory1/1, AND2/2
  Switch1/1 -> Switch/3
  enable_RAM_indexing/1 -> AND2/1, Memory2/1, find_first_one_pos/Enable, find_next_chip_rollmap/Enable, RAM_address_channel_data/Enable, enable_source_chip_transmission/Enable
  FIFO_write_to/1 -> enable_RAM_indexing/1
  find_next_chip_rollmap/1(bit_masked) -> Compare To Constant5/1, Memory/1  "next_chip_rollmap"
  data_stream_enable/1 -> Switch/1, Switch1/1
  Compare To Constant1/1 -> Switch/2
  Switch/1 -> find_first_one_pos/1(In1), find_next_chip_rollmap/1(curr_chip_rollmap)  "curr_chip_rollmap"
  InputState/1 -> Compare To Constant3/1, Compare To Constant4/1, Compare To Constant6/1, Compare To Constant2/1, Compare To Constant1/1  "input state"

== system gm_CustArch_v5_vnl/cust_architecture_vnl/output_interpret/Interpret_to_RAM_output/get_enabled_timings /find_next_chip_rollmap ==
  note: bit rotation --> circular rotation of the data_stream_enable 8-bit string
      |
      | Example: data_stream_enable == 01001000
      | right rotation length 1 --> 00100100
      | right rotation length 3 --> 10000100
  note: this is to identify the next chip for decoding process
  In1 : Inport
  Trigger : TriggerPort  VariantControl=Variant
  Bit Rotate : hdlsllib/Logic and Bit Operations/Bit Rotate  mode=Rotate Right  N=1
      settings: SourceProductBaseCode=SL
  Out1 : Outport  InitialOutput=0  VectorParamsAs1DForOutWhenUnconnected=off
  wires:
  Bit Rotate/1 -> Out1/1
  In1/1 -> Bit Rotate/1

== system gm_CustArch_v5_vnl/cust_architecture_vnl/output_interpret/Interpret_to_RAM_output/get_enabled_timings /reading_address ==
  note: this is the ugliest thing ever--- but it works.. so far so good
  "counter " : Inport
  data_stream_en : Inport  Port=2
  Bit Rotate : hdlsllib/Logic and Bit Operations/Bit Rotate  mode=Rotate Right  N=1
      settings: SourceProductBaseCode=SL
  Bit Rotate1 : hdlsllib/Logic and Bit Operations/Bit Rotate  mode=Rotate Right  N=2
      settings: SourceProductBaseCode=SL
  Bit Rotate2 : hdlsllib/Logic and Bit Operations/Bit Rotate  mode=Rotate Right  N=3
      settings: SourceProductBaseCode=SL
  Bit Rotate3 : hdlsllib/Logic and Bit Operations/Bit Rotate  mode=Rotate Right  N=4
      settings: SourceProductBaseCode=SL
  Bit Rotate4 : hdlsllib/Logic and Bit Operations/Bit Rotate  mode=Rotate Right  N=5
      settings: SourceProductBaseCode=SL
  Bit Rotate5 : hdlsllib/Logic and Bit Operations/Bit Rotate  mode=Rotate Right  N=6
      settings: SourceProductBaseCode=SL
  Bit Rotate6 : hdlsllib/Logic and Bit Operations/Bit Rotate  mode=Rotate Right  N=7
      settings: SourceProductBaseCode=SL
  Bit Slice : hdlsllib/Logic and Bit Operations/Bit Slice  lidx=0  ridx=0
      settings: SourceProductBaseCode=SL
  Compare To Constant : simulink/Logic and Bit Operations/Compare To Constant  relop===  const=0  OutDataTypeStr=boolean
  Compare To Constant1 : simulink/Logic and Bit Operations/Compare To Constant  relop===  const=1  OutDataTypeStr=boolean
  Compare To Constant2 : simulink/Logic and Bit Operations/Compare To Constant  relop===  const=2  OutDataTypeStr=boolean
  Compare To Constant3 : simulink/Logic and Bit Operations/Compare To Constant  relop===  const=3  OutDataTypeStr=boolean
  Compare To Constant4 : simulink/Logic and Bit Operations/Compare To Constant  relop===  const=4  OutDataTypeStr=boolean
  Compare To Constant5 : simulink/Logic and Bit Operations/Compare To Constant  relop===  const=5  OutDataTypeStr=boolean
  Compare To Constant6 : simulink/Logic and Bit Operations/Compare To Constant  relop===  const=6  OutDataTypeStr=boolean
  Compare To Constant7 : simulink/Logic and Bit Operations/Compare To Constant  relop===  const=7  OutDataTypeStr=boolean
  Constant : Constant  Value=0  OutDataTypeStr=uint8  SampleTime=-1
  Switch{,1..7} (8 alike) : Switch  Criteria=u2 > Threshold
  source_device_en : Outport  VectorParamsAs1DForOutWhenUnconnected=off
  source_device : Outport  Port=2  VectorParamsAs1DForOutWhenUnconnected=off
  wires:
  Bit Slice/1 -> source_device_en/1
  Switch/1 -> Bit Slice/1
  data_stream_en/1 -> Bit Rotate6/1, Bit Rotate5/1, Bit Rotate4/1, Bit Rotate3/1, Bit Rotate2/1, Bit Rotate1/1, Bit Rotate/1, Switch/1
  Switch2/1 -> Switch1/3
  Constant/1 -> Switch7/3
  Bit Rotate6/1 -> Switch7/1
  Switch7/1 -> Switch6/3
  Compare To Constant7/1 -> Switch7/2
  Bit Rotate5/1 -> Switch6/1
  Switch6/1 -> Switch5/3
  Compare To Constant6/1 -> Switch6/2
  Switch5/1 -> Switch4/3
  Bit Rotate4/1 -> Switch5/1
  Compare To Constant5/1 -> Switch5/2
  Bit Rotate3/1 -> Switch4/1
  Switch4/1 -> Switch3/3
  Compare To Constant4/1 -> Switch4/2
  Bit Rotate2/1 -> Switch3/1
  Switch3/1 -> Switch2/3
  Compare To Constant3/1 -> Switch3/2
  Bit Rotate1/1 -> Switch2/1
  Compare To Constant2/1 -> Switch2/2
  Switch1/1 -> Switch/3
  "counter "/1 -> source_device/1, Compare To Constant/1, Compare To Constant1/1, Compare To Constant2/1, Compare To Constant3/1, Compare To Constant4/1, Compare To Constant5/1, Compare To Constant6/1, Compare To Constant7/1
  Bit Rotate/1 -> Switch1/1
  Compare To Constant1/1 -> Switch1/2
  Compare To Constant/1 -> Switch/2

== system gm_CustArch_v5_vnl/cust_architecture/input_interpret_store_retrieve/Interpret_to_RAM_input/interpret incoming data/get_sources_and_RAM_addresses/RAM_address_channel_data ==
  source_device : Inport  OutDataTypeStr=uint8  PortDimensions=1  SampleTime=1
  dev_output : Inport  Port=2  OutDataTypeStr=uint8  PortDimensions=1  SampleTime=1
  Enable : EnablePort  OutDataTypeStr=boolean
  Bit Concat : hdlsllib/Logic and Bit Operations/Bit Concat  numInputs=2
  Bit Slice : hdlsllib/Logic and Bit Operations/Bit Slice  lidx=double(4)  ridx=double(0)
      settings: SourceProductBaseCode=SL
  Bit Slice1 : hdlsllib/Logic and Bit Operations/Bit Slice  lidx=double(2)  ridx=double(0)
      settings: SourceProductBaseCode=SL
  source_channel_0_159 : Outport  InitialOutput=0  VectorParamsAs1DForOutWhenUnconnected=off
  wires:
  Bit Slice1/1 -> Bit Concat/2
  Bit Slice/1 -> Bit Concat/1
  Bit Concat/1 -> source_channel_0_159/1
  dev_output/1 -> Bit Slice/1
  source_device/1 -> Bit Slice1/1

== system gm_CustArch_v5_vnl/cust_architecture/input_interpret_store_retrieve/Interpret_to_RAM_input/interpret incoming data/get_sources_and_RAM_addresses/enable_source_chip_transmission ==
  In1 : Inport  OutDataTypeStr=uint8  PortDimensions=1  SampleTime=1
  Enable : EnablePort  OutDataTypeStr=boolean
  Out1 : Outport  InitialOutput=0  VectorParamsAs1DForOutWhenUnconnected=off
  wires:
  In1/1 -> Out1/1

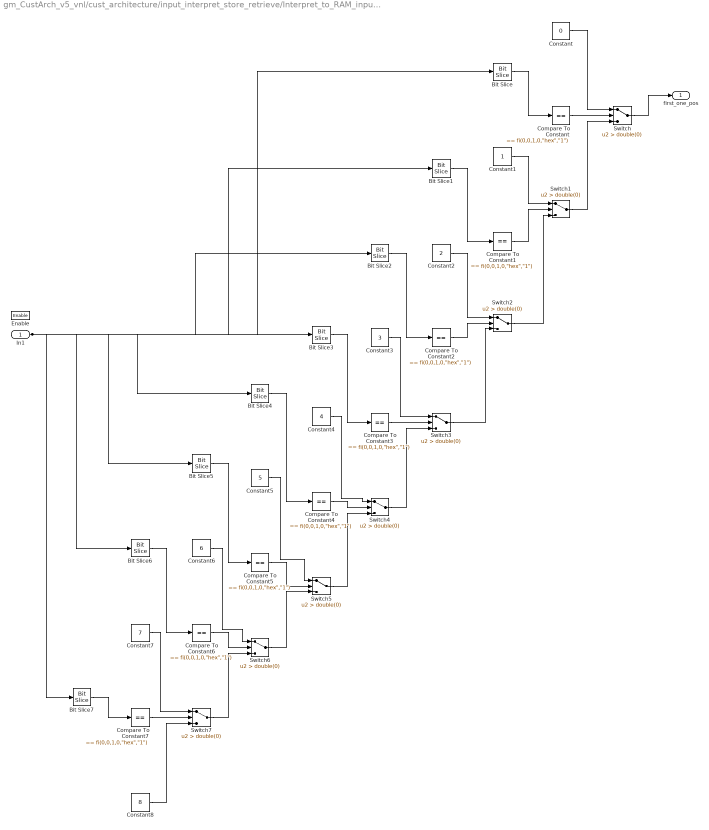
== system gm_CustArch_v5_vnl/cust_architecture/input_interpret_store_retrieve/Interpret_to_RAM_input/interpret incoming data/get_sources_and_RAM_addresses/find_first_one_pos ==
  In1 : Inport  OutDataTypeStr=uint8  PortDimensions=1  SampleTime=1
  Enable : EnablePort  OutDataTypeStr=boolean
  Bit Slice : hdlsllib/Logic and Bit Operations/Bit Slice  lidx=double(0)  ridx=double(0)
      settings: SourceProductBaseCode=SL
  Bit Slice1 : hdlsllib/Logic and Bit Operations/Bit Slice  lidx=double(1)  ridx=double(1)
      settings: SourceProductBaseCode=SL
  Bit Slice2 : hdlsllib/Logic and Bit Operations/Bit Slice  lidx=double(2)  ridx=double(2)
      settings: SourceProductBaseCode=SL
  Bit Slice3 : hdlsllib/Logic and Bit Operations/Bit Slice  lidx=double(3)  ridx=double(3)
      settings: SourceProductBaseCode=SL
  Bit Slice4 : hdlsllib/Logic and Bit Operations/Bit Slice  lidx=double(4)  ridx=double(4)
      settings: SourceProductBaseCode=SL
  Bit Slice5 : hdlsllib/Logic and Bit Operations/Bit Slice  lidx=double(5)  ridx=double(5)
      settings: SourceProductBaseCode=SL
  Bit Slice6 : hdlsllib/Logic and Bit Operations/Bit Slice  lidx=double(6)  ridx=double(6)
      settings: SourceProductBaseCode=SL
  Bit Slice7 : hdlsllib/Logic and Bit Operations/Bit Slice  lidx=double(7)  ridx=double(7)
      settings: SourceProductBaseCode=SL
  Compare To Constant{,1..7} (8 alike) : simulink/Logic and Bit Operations/Compare To Constant  relop===  const="fi(0,0,1,0,\"hex\",\"1\")"  OutDataTypeStr=boolean
  Constant : Constant  Value=0  OutDataTypeStr=uint8  SampleTime=1
  Constant1 : Constant  OutDataTypeStr=uint8  SampleTime=1
  Constant2 : Constant  Value=2  OutDataTypeStr=uint8  SampleTime=1
  Constant3 : Constant  Value=3  OutDataTypeStr=uint8  SampleTime=1
  Constant4 : Constant  Value=4  OutDataTypeStr=uint8  SampleTime=1
  Constant5 : Constant  Value=5  OutDataTypeStr=uint8  SampleTime=1
  Constant6 : Constant  Value=6  OutDataTypeStr=uint8  SampleTime=1
  Constant7 : Constant  Value=7  OutDataTypeStr=uint8  SampleTime=1
  Constant8 : Constant  Value=8  OutDataTypeStr=uint8  SampleTime=1
  Switch{,1..7} (8 alike) : Switch  Criteria=u2 > Threshold  Threshold=double(0)  OutDataTypeStr=uint8  SampleTime=1
  first_one_pos : Outport  InitialOutput=0  VectorParamsAs1DForOutWhenUnconnected=off
  wires:
  Switch7/1 -> Switch6/3
  Switch6/1 -> Switch5/3
  Switch5/1 -> Switch4/3
  Switch4/1 -> Switch3/3
  Switch3/1 -> Switch2/3
  Switch2/1 -> Switch1/3
  Switch1/1 -> Switch/3
  Switch/1 -> first_one_pos/1
  Constant8/1 -> Switch7/3
  Constant7/1 -> Switch7/1
  Constant6/1 -> Switch6/1
  Constant5/1 -> Switch5/1
  Constant4/1 -> Switch4/1
  Constant3/1 -> Switch3/1
  Constant2/1 -> Switch2/1
  Constant1/1 -> Switch1/1
  Constant/1 -> Switch/1
  Compare To Constant7/1 -> Switch7/2
  Compare To Constant6/1 -> Switch6/2
  Compare To Constant5/1 -> Switch5/2
  Compare To Constant4/1 -> Switch4/2
  Compare To Constant3/1 -> Switch3/2
  Compare To Constant2/1 -> Switch2/2
  Compare To Constant1/1 -> Switch1/2
  Compare To Constant/1 -> Switch/2
  Bit Slice7/1 -> Compare To Constant7/1
  Bit Slice6/1 -> Compare To Constant6/1
  Bit Slice5/1 -> Compare To Constant5/1
  Bit Slice4/1 -> Compare To Constant4/1
  Bit Slice3/1 -> Compare To Constant3/1
  Bit Slice2/1 -> Compare To Constant2/1
  Bit Slice1/1 -> Compare To Constant1/1
  Bit Slice/1 -> Compare To Constant/1
  In1/1 -> Bit Slice/1, Bit Slice1/1, Bit Slice2/1, Bit Slice3/1, Bit Slice4/1, Bit Slice5/1, Bit Slice6/1, Bit Slice7/1

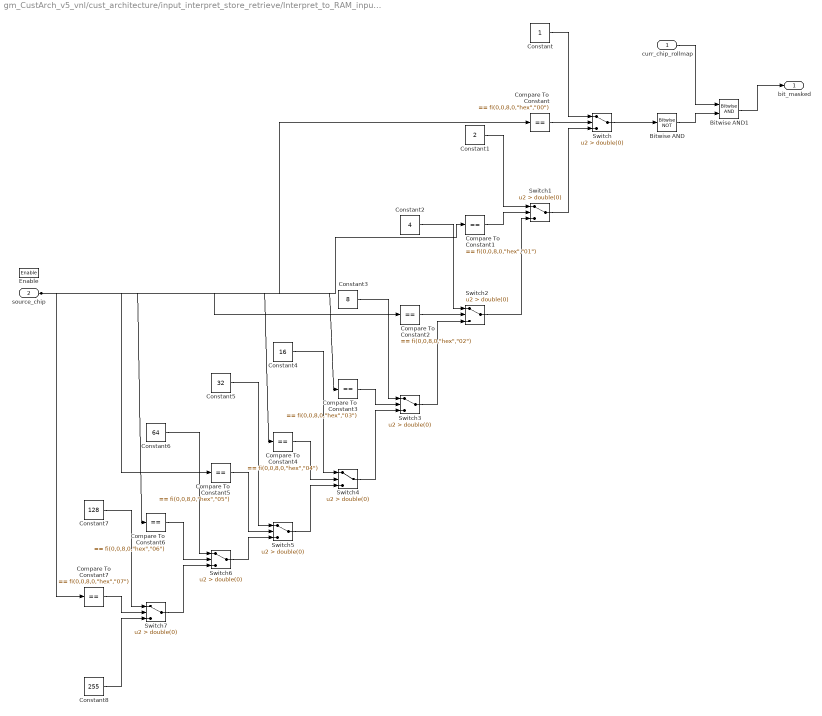
== system gm_CustArch_v5_vnl/cust_architecture/input_interpret_store_retrieve/Interpret_to_RAM_input/interpret incoming data/get_sources_and_RAM_addresses/find_next_chip_rollmap ==
  curr_chip_rollmap : Inport  OutDataTypeStr=uint8  PortDimensions=1  SampleTime=1
  source_chip : Inport  Port=2  OutDataTypeStr=uint8  PortDimensions=1  SampleTime=1
  Enable : EnablePort  OutDataTypeStr=boolean
  Bitwise AND : simulink/Logic and Bit Operations/Bitwise Operator  logicop=NOT  UseBitMask=off  BitMask=double(0)  BitMaskRealWorld=Real World Value
  Bitwise AND1 : simulink/Logic and Bit Operations/Bitwise Operator  logicop=AND  UseBitMask=off  NumInputPorts=2  BitMask=double(0)  BitMaskRealWorld=Real World Value
  Compare To Constant : simulink/Logic and Bit Operations/Compare To Constant  relop===  const="fi(0,0,8,0,\"hex\",\"00\")"  OutDataTypeStr=boolean
  Compare To Constant1 : simulink/Logic and Bit Operations/Compare To Constant  relop===  const="fi(0,0,8,0,\"hex\",\"01\")"  OutDataTypeStr=boolean
  Compare To Constant2 : simulink/Logic and Bit Operations/Compare To Constant  relop===  const="fi(0,0,8,0,\"hex\",\"02\")"  OutDataTypeStr=boolean
  Compare To Constant3 : simulink/Logic and Bit Operations/Compare To Constant  relop===  const="fi(0,0,8,0,\"hex\",\"03\")"  OutDataTypeStr=boolean
  Compare To Constant4 : simulink/Logic and Bit Operations/Compare To Constant  relop===  const="fi(0,0,8,0,\"hex\",\"04\")"  OutDataTypeStr=boolean
  Compare To Constant5 : simulink/Logic and Bit Operations/Compare To Constant  relop===  const="fi(0,0,8,0,\"hex\",\"05\")"  OutDataTypeStr=boolean
  Compare To Constant6 : simulink/Logic and Bit Operations/Compare To Constant  relop===  const="fi(0,0,8,0,\"hex\",\"06\")"  OutDataTypeStr=boolean
  Compare To Constant7 : simulink/Logic and Bit Operations/Compare To Constant  relop===  const="fi(0,0,8,0,\"hex\",\"07\")"  OutDataTypeStr=boolean
  Constant : Constant  OutDataTypeStr=uint8  SampleTime=1
  Constant1 : Constant  Value=2  OutDataTypeStr=uint8  SampleTime=1
  Constant2 : Constant  Value=4  OutDataTypeStr=uint8  SampleTime=1
  Constant3 : Constant  Value=8  OutDataTypeStr=uint8  SampleTime=1
  Constant4 : Constant  Value=16  OutDataTypeStr=uint8  SampleTime=1
  Constant5 : Constant  Value=32  OutDataTypeStr=uint8  SampleTime=1
  Constant6 : Constant  Value=64  OutDataTypeStr=uint8  SampleTime=1
  Constant7 : Constant  Value=128  OutDataTypeStr=uint8  SampleTime=1
  Constant8 : Constant  Value=255  OutDataTypeStr=uint8  SampleTime=1
  Switch{,1..7} (8 alike) : Switch  Criteria=u2 > Threshold  Threshold=double(0)  OutDataTypeStr=uint8  SampleTime=1
  bit_masked : Outport  InitialOutput=0  VectorParamsAs1DForOutWhenUnconnected=off
  wires:
  Switch7/1 -> Switch6/3
  Switch6/1 -> Switch5/3
  Switch5/1 -> Switch4/3
  Switch4/1 -> Switch3/3
  Switch3/1 -> Switch2/3
  Switch2/1 -> Switch1/3
  Switch1/1 -> Switch/3
  Switch/1 -> Bitwise AND/1
  Constant8/1 -> Switch7/3
  Constant7/1 -> Switch7/1
  Constant6/1 -> Switch6/1
  Constant5/1 -> Switch5/1
  Constant4/1 -> Switch4/1
  Constant3/1 -> Switch3/1
  Constant2/1 -> Switch2/1
  Constant1/1 -> Switch1/1
  Constant/1 -> Switch/1
  Compare To Constant7/1 -> Switch7/2
  Compare To Constant6/1 -> Switch6/2
  Compare To Constant5/1 -> Switch5/2
  Compare To Constant4/1 -> Switch4/2
  Compare To Constant3/1 -> Switch3/2
  Compare To Constant2/1 -> Switch2/2
  Compare To Constant1/1 -> Switch1/2
  Compare To Constant/1 -> Switch/2
  Bitwise AND1/1 -> bit_masked/1
  Bitwise AND/1 -> Bitwise AND1/2
  source_chip/1 -> Compare To Constant/1, Compare To Constant1/1, Compare To Constant2/1, Compare To Constant3/1, Compare To Constant4/1, Compare To Constant5/1, Compare To Constant6/1, Compare To Constant7/1
  curr_chip_rollmap/1 -> Bitwise AND1/1

== system gm_CustArch_v5_vnl/cust_architecture_vnl/input_interpret_store_retrieve/Interpret_to_RAM_input/interpret incoming data/get_sources_and_RAM_addresses/RAM_address_channel_data ==
  note: channel data address codification
      | according to this table
  source_device : Inport
  dev_output : Inport  Port=2
  Enable : EnablePort
  Bit Concat : hdlsllib/Logic and Bit Operations/Bit Concat  numInputs=2  mask(Bit Concat){}
      mask Display: image('C:\Users\diflo\OneDrive - Fondazione Istituto Italiano Tecnologia\Progetto MathWorks\Project\Documentation\Images\Simulink\source_channel_0_159.png'); % Use "Edit Image" on toolstrip to change.
  Bit Slice : hdlsllib/Logic and Bit Operations/Bit Slice  lidx=4  ridx=0
      settings: SourceProductBaseCode=SL
  Bit Slice1 : hdlsllib/Logic and Bit Operations/Bit Slice  lidx=2  ridx=0
      settings: SourceProductBaseCode=SL
  source_channel_0_159 : Outport  InitialOutput=0  VectorParamsAs1DForOutWhenUnconnected=off
  wires:
  dev_output/1 -> Bit Slice/1
  Bit Concat/1 -> source_channel_0_159/1  "source_channel_0_159"
  Bit Slice1/1 -> Bit Concat/2
  Bit Slice/1 -> Bit Concat/1
  source_device/1 -> Bit Slice1/1

== system gm_CustArch_v5_vnl/cust_architecture_vnl/input_interpret_store_retrieve/Interpret_to_RAM_input/interpret incoming data/get_sources_and_RAM_addresses/enable_source_chip_transmission ==
  In1 : Inport
  Enable : EnablePort
  Out1 : Outport  InitialOutput=0  VectorParamsAs1DForOutWhenUnconnected=off
  wires:
  In1/1 -> Out1/1

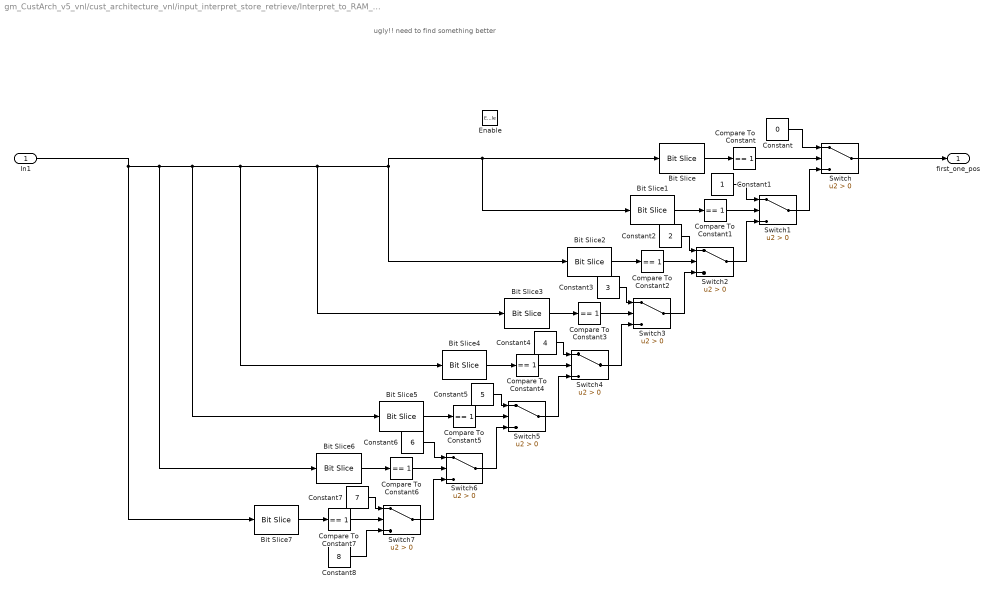
== system gm_CustArch_v5_vnl/cust_architecture_vnl/input_interpret_store_retrieve/Interpret_to_RAM_input/interpret incoming data/get_sources_and_RAM_addresses/find_first_one_pos ==
  note: ugly!! need to find something better
  In1 : Inport
  Enable : EnablePort
  Bit Slice : hdlsllib/Logic and Bit Operations/Bit Slice  lidx=0  ridx=0
      settings: SourceProductBaseCode=SL
  Bit Slice1 : hdlsllib/Logic and Bit Operations/Bit Slice  lidx=1  ridx=1
      settings: SourceProductBaseCode=SL
  Bit Slice2 : hdlsllib/Logic and Bit Operations/Bit Slice  lidx=2  ridx=2
      settings: SourceProductBaseCode=SL
  Bit Slice3 : hdlsllib/Logic and Bit Operations/Bit Slice  lidx=3  ridx=3
      settings: SourceProductBaseCode=SL
  Bit Slice4 : hdlsllib/Logic and Bit Operations/Bit Slice  lidx=4  ridx=4
      settings: SourceProductBaseCode=SL
  Bit Slice5 : hdlsllib/Logic and Bit Operations/Bit Slice  lidx=5  ridx=5
      settings: SourceProductBaseCode=SL
  Bit Slice6 : hdlsllib/Logic and Bit Operations/Bit Slice  lidx=6  ridx=6
      settings: SourceProductBaseCode=SL
  Bit Slice7 : hdlsllib/Logic and Bit Operations/Bit Slice  lidx=7  ridx=7
      settings: SourceProductBaseCode=SL
  Compare To Constant{,1..7} (8 alike) : simulink/Logic and Bit Operations/Compare To Constant  relop===  const=1  OutDataTypeStr=boolean
  Constant : Constant  Value=0  OutDataTypeStr=uint8  SampleTime=-1
  Constant1 : Constant  OutDataTypeStr=uint8  SampleTime=-1
  Constant2 : Constant  Value=2  OutDataTypeStr=uint8  SampleTime=-1
  Constant3 : Constant  Value=3  OutDataTypeStr=uint8  SampleTime=-1
  Constant4 : Constant  Value=4  OutDataTypeStr=uint8  SampleTime=-1
  Constant5 : Constant  Value=5  OutDataTypeStr=uint8  SampleTime=-1
  Constant6 : Constant  Value=6  OutDataTypeStr=uint8  SampleTime=-1
  Constant7 : Constant  Value=7  OutDataTypeStr=uint8  SampleTime=-1
  Constant8 : Constant  Value=8  OutDataTypeStr=uint8  SampleTime=-1
  Switch{,1..7} (8 alike) : Switch  Criteria=u2 > Threshold
  first_one_pos : Outport  InitialOutput=0  VectorParamsAs1DForOutWhenUnconnected=off
  wires:
  In1/1 -> Bit Slice/1, Bit Slice1/1, Bit Slice2/1, Bit Slice3/1, Bit Slice4/1, Bit Slice5/1, Bit Slice6/1, Bit Slice7/1
  Constant8/1 -> Switch7/3
  Constant7/1 -> Switch7/1
  Constant6/1 -> Switch6/1
  Constant5/1 -> Switch5/1
  Constant4/1 -> Switch4/1
  Constant3/1 -> Switch3/1
  Constant2/1 -> Switch2/1
  Constant1/1 -> Switch1/1
  Constant/1 -> Switch/1
  Bit Slice7/1 -> Compare To Constant7/1
  Compare To Constant7/1 -> Switch7/2
  Switch7/1 -> Switch6/3
  Switch6/1 -> Switch5/3
  Compare To Constant6/1 -> Switch6/2
  Bit Slice6/1 -> Compare To Constant6/1
  Switch5/1 -> Switch4/3
  Compare To Constant5/1 -> Switch5/2
  Bit Slice5/1 -> Compare To Constant5/1
  Compare To Constant4/1 -> Switch4/2
  Bit Slice4/1 -> Compare To Constant4/1
  Switch4/1 -> Switch3/3
  Switch3/1 -> Switch2/3
  Compare To Constant3/1 -> Switch3/2
  Bit Slice3/1 -> Compare To Constant3/1
  Switch2/1 -> Switch1/3
  Compare To Constant2/1 -> Switch2/2
  Bit Slice2/1 -> Compare To Constant2/1
  Compare To Constant1/1 -> Switch1/2
  Switch1/1 -> Switch/3
  Bit Slice1/1 -> Compare To Constant1/1
  Switch/1 -> first_one_pos/1
  Bit Slice/1 -> Compare To Constant/1
  Compare To Constant/1 -> Switch/2
